simulink model "Trans"  (R2018b)
settings: Solver=FixedStepAuto  StartTime=0.0  StopTime=5000  FixedStep=10  RelTol=1e-3
values from neighbouring files (symbols this model uses):
  dt = 500    [script1.m]
  dTg = 0    [script1.m]
  dTkz = 0    [script1.m]
  dTzew = 0    [script1.m]
  L11 = [Cp0*CVp, Cp0*(kp+k2)]    [script1.m]
  L12 = [CVp*k1, k1*(k2+kp)]    [script1.m]
  L13 = [k2*kp]    [script1.m]
  L21 = [Cp0*kp]    [script1.m]
  L22 = [k1*kp]    [script1.m]
  L23 = [CVw*k2 (k2*Cp0+k1*k2+k2*kp)]    [script1.m]
  M = [CVw * CVp, CVw*kp + CVw*k2 + Cp0*CVp + CVp*k1 + CVp*kp, (kp+k2)*(Cp0) + k1*kp + k1*k2 + kp*k2]    [script1.m]
  Tp0 = (kp * Twew0 + k2 * Tg0) / (k2 + kp)    (= 10)    [script1.m]
  Twew0 = (Cp0 * Tkz0 + k1 * Tzew0 + k2 * kp * Tg0 / (k2 + kp)) / (Cp0 + k1 + kp - kp * kp / (k2 + kp))    (= 20)    [script1.m]
settings Model: Creator=wojciechkonury  LastModifiedBy=wojciechkonury

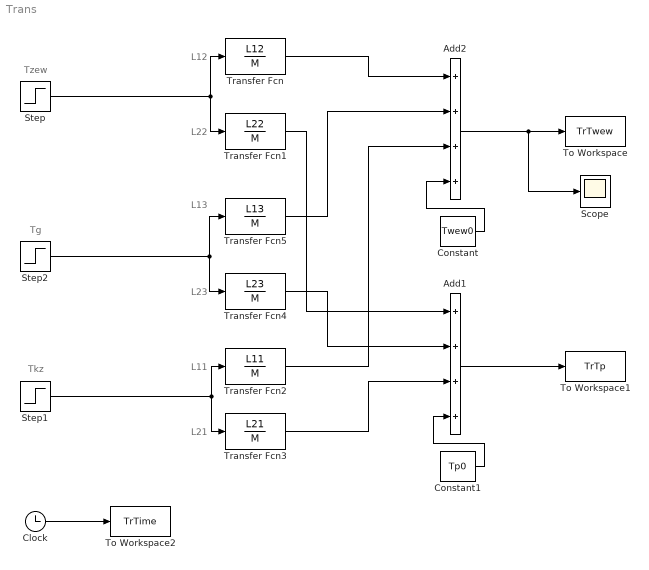
== system Trans ==
  note: L22
  note: L12
  note: L23
  note: L13
  note: L21
  note: L11
  note: Tkz
  note: Tg
  note: Tzew
  Add1 : Sum  Inputs=++++
  Add2 : Sum  Inputs=++++
  Clock : Clock
  Constant : Constant  Value=Twew0
  Constant1 : Constant  Value=Tp0
  Scope : Scope
  Step : Step  Time=dt  After=dTzew  SampleTime=0
  Step1 : Step  Time=dt  After=dTkz  SampleTime=0
  Step2 : Step  Time=dt  After=dTg  SampleTime=0
  To Workspace : ToWorkspace  VariableName=TrTwew  SampleTime=-1
  To Workspace1 : ToWorkspace  VariableName=TrTp  SampleTime=-1
  To Workspace2 : ToWorkspace  VariableName=TrTime  SampleTime=-1
  Transfer Fcn : TransferFcn  Numerator=L12  Denominator=M
  Transfer Fcn1 : TransferFcn  Numerator=L22  Denominator=M
  Transfer Fcn2 : TransferFcn  Numerator=L11  Denominator=M
  Transfer Fcn3 : TransferFcn  Numerator=L21  Denominator=M
  Transfer Fcn4 : TransferFcn  Numerator=L23  Denominator=M
  Transfer Fcn5 : TransferFcn  Numerator=L13  Denominator=M
  wires:
  Step1/1 -> Transfer Fcn3/1, Transfer Fcn2/1
  Step2/1 -> Transfer Fcn5/1, Transfer Fcn4/1
  Step/1 -> Transfer Fcn/1, Transfer Fcn1/1
  Transfer Fcn2/1 -> Add2/3
  Transfer Fcn5/1 -> Add2/2
  Transfer Fcn/1 -> Add2/1
  Transfer Fcn3/1 -> Add1/3
  Transfer Fcn4/1 -> Add1/2
  Transfer Fcn1/1 -> Add1/1
  Constant/1 -> Add2/4
  Constant1/1 -> Add1/4
  Add1/1 -> To Workspace1/1
  Add2/1 -> Scope/1, To Workspace/1
  Clock/1 -> To Workspace2/1
